simulink model "board_unspecific_serial"  (R2015a)
settings: Solver=FixedStepDiscrete  SolverMode=SingleTasking  StartTime=0.0  StopTime=10.0  FixedStep=1e-3  RelTol=1e-3
libraries: mbed_lib x3
settings Model: Creator=oh  LastModifiedBy=oh
settings OptimizationCC: OptimizeModelRefInitCode=on  LifeSpan=1
settings HardwareCC: ProdLargestAtomicInteger=Long  ProdLargestAtomicFloat=Double  ProdEndianess=LittleEndian  ProdHWDeviceType=ARM Compatible->ARM Cortex
settings RTWCC: SystemTargetFile=mbed.tlc  TemplateMakefile=mbed.tmf  Description=Mbed Target (Embedded Target)  TargetLang=C++
settings CodeAppCC: IgnoreCustomStorageClasses=off
settings STFCustomTargetCC: CombineOutputUpdateFcns=on  SupportContinuousTime=off  SupportVariableSizeSignals=off  SystemTargetFile=mbed.tlc
settings ERTTargetCC: SupportContinuousTime=off  SupportVariableSizeSignals=off  ERTCustomFileTemplate=mbed_file_process.tlc

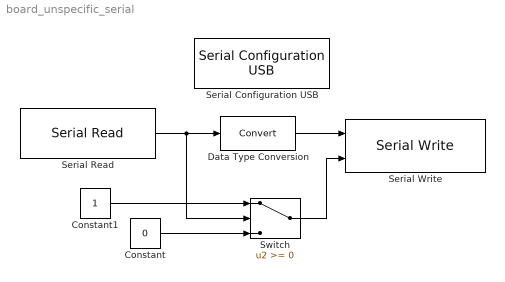
== system board_unspecific_serial ==
  Constant : Constant  Value=0  OutDataTypeStr=uint32
  Constant1 : Constant  OutDataTypeStr=uint32
  Data Type Conversion : DataTypeConversion
  Serial Configuration USB : mbed_lib/Serial/Serial Configuration USB  BaudRate=9600
  Serial Read : mbed_lib/Serial/Serial Read  SerialPort=0  SampleTime=-1
  Serial Write : mbed_lib/Serial/Serial Write  SerialPort=0  numData=on  SampleTime=-1
  Switch : Switch
  wires:
  Serial Read/1 -> Switch/2, Data Type Conversion/1
  Data Type Conversion/1 -> Serial Write/1
  Constant1/1 -> Switch/1
  Constant/1 -> Switch/3
  Switch/1 -> Serial Write/2
